simulink model "ex3_sim1"  (R2018b)
settings: Solver=ode45  StartTime=0.0  StopTime=4  MaxStep=0.01  RelTol=1e-3
undefined symbols (not defined in the file): Ad, Ar, denH, denP, denQ, kp, numH, numP, numQ, t0d, t0r
settings Model: Creator=riccardo  LastModifiedBy=riccardo

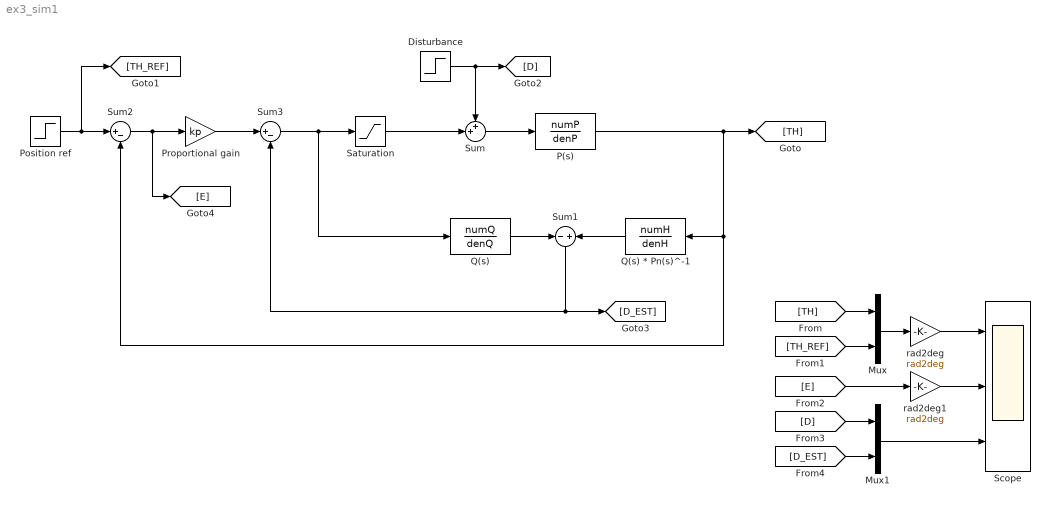
== system ex3_sim1 ==
  Disturbance : Step  Time=t0d  After=Ad  SampleTime=0
  Mux : Mux  Inputs=2
  Mux1 : Mux  Inputs=2
  P(s) : TransferFcn  Numerator=numP  Denominator=denP
  Position ref : Step  Time=t0r  After=Ar  SampleTime=0
  Proportional gain : Gain  Gain=kp
  Q(s) : TransferFcn  Numerator=numQ  Denominator=denQ
  Q(s) * Pn(s)^-1 : TransferFcn  Numerator=numH  Denominator=denH
  Saturation : Saturate  UpperLimit=10  LowerLimit=-10
  Scope : Scope  NumInputPorts=3
  Sum : Sum  Inputs=++|
  Sum1 : Sum  Inputs=-+
  Sum2 : Sum  Inputs=|+-
  Sum3 : Sum  Inputs=|+-
  rad2deg : Gain  Gain=rad2deg
  rad2deg1 : Gain  Gain=rad2deg
  wires:
  Sum/1 -> P(s)/1
  P(s)/1 -> [TH], Q(s) * Pn(s)^-1/1, Sum2/2
  Q(s)/1 -> Sum1/1
  Q(s) * Pn(s)^-1/1 -> Sum1/2
  Saturation/1 -> Sum/2
  Sum2/1 -> [E], Proportional gain/1
  Position ref/1 -> [TH_REF], Sum2/1
  Disturbance/1 -> [D], Sum/1
  Sum3/1 -> Q(s)/1, Saturation/1
  Proportional gain/1 -> Sum3/1
  Sum1/1 -> Sum3/2, [D_EST]
  Mux/1 -> rad2deg/1
  [TH] -> Mux/1
  [TH_REF] -> Mux/2
  rad2deg/1 -> Scope/1
  [E] -> rad2deg1/1
  Mux1/1 -> Scope/3
  [D] -> Mux1/1
  [D_EST] -> Mux1/2
  rad2deg1/1 -> Scope/2
